simulink model "LIPModel"  (R2016b)
settings: Solver=FixedStepAuto  StartTime=0.0  StopTime=80  FixedStep=0.02  RelTol=1e-3  EnableMultiTasking=on
libraries: powerlib_meascontrol x2
settings Model: Creator=mdai3  LastModifiedBy=WZE7470
settings DataIOCC: ReturnWorkspaceOutputs=on
settings SFSimCC: SimUseLocalCustomCode=on
settings RTWCC: RTWUseLocalCustomCode=on

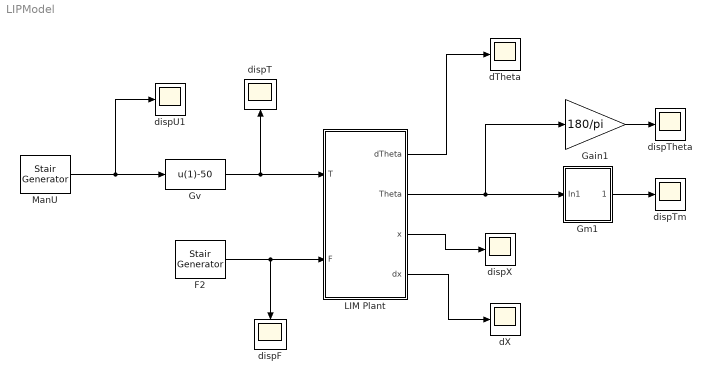
== system LIPModel ==
  F2 : powerlib_meascontrol/Pulse & Signal Generators/Stair Generator  t=[0, 5, 35, 65]  e=[0, 5, -5, 0]  Ts=0
  Gain1 : Gain  Gain=180/pi
  Gm1 : Subsystem  mask(TF with U0, Y0){Num=[1], Den=[0.2 1], U0=-pi/2, Y0=-pi/2}
      mask help: TF with Initial U0, Y0
      mask Display: dpoly(Num,Den,'s');
  Gv : Fcn  Expr=u(1)-50
  LIM Plant : Subsystem  mask(LIP Model){x0=0, Theta0=-pi/2}
      mask prompts: x0 "Initial Position, x0"; Theta0 "Initial Angle"
  ManU : powerlib_meascontrol/Pulse & Signal Generators/Stair Generator  t=[0, 10, 15, 20]  e=[50, 51, 49, 50]  Ts=0
  dTheta : Scope
  dX : Scope
  dispF : Scope
  dispT : Scope
  dispTheta : Scope
  dispTm : Scope
  dispU1 : Scope
  dispX : Scope
  wires:
  ManU/1 -> dispU1/1, Gv/1
  F2/1 -> LIM Plant/2(F), dispF/1
  Gain1/1 -> dispTheta/1
  LIM Plant/2(Theta) -> Gm1/1(In1), Gain1/1
  Gv/1 -> dispT/1, LIM Plant/1(T)
  LIM Plant/1(dTheta) -> dTheta/1
  LIM Plant/3(x) -> dispX/1
  LIM Plant/4(dx) -> dX/1
  Gm1/1(Out1) -> dispTm/1

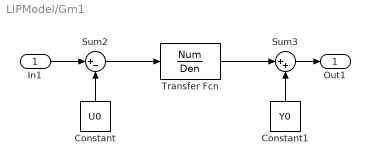
== system LIPModel/Gm1 ==
  In1 : Inport
  Constant : Constant  Value=U0
  Constant1 : Constant  Value=Y0
  Sum2 : Sum  Inputs=|+-  SaturateOnIntegerOverflow=on
  Sum3 : Sum  Inputs=|++  SaturateOnIntegerOverflow=on
  Transfer Fcn : TransferFcn  Numerator=Num  Denominator=Den
  Out1 : Outport
  wires:
  Constant/1 -> Sum2/2
  Constant1/1 -> Sum3/2
  Transfer Fcn/1 -> Sum3/1
  In1/1 -> Sum2/1
  Sum3/1 -> Out1/1
  Sum2/1 -> Transfer Fcn/1

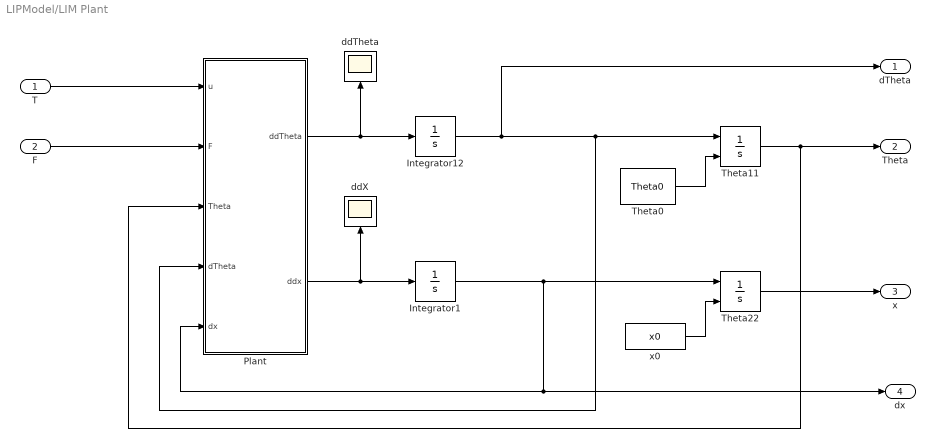
== system LIPModel/LIM Plant ==
  T : Inport
  F : Inport  Port=2
  Integrator1 : Integrator  UpperSaturationLimit=1  LowerSaturationLimit=-1
  Integrator12 : Integrator  UpperSaturationLimit=1  LowerSaturationLimit=-1
  Plant : MATLAB Function  TreatAsAtomicUnit=on
  Theta0 : Constant  Value=Theta0
  Theta11 : Integrator  InitialConditionSource=external  LimitOutput=on  UpperSaturationLimit=pi  LowerSaturationLimit=-pi
  Theta22 : Integrator  InitialConditionSource=external  LimitOutput=on  LowerSaturationLimit=0
  ddTheta : Scope
  ddX : Scope
  x0 : Constant  Value=x0
  dTheta : Outport
  Theta : Outport  Port=2
  x : Outport  Port=3
  dx : Outport  Port=4
  wires:
  F/1 -> Plant/2(F)
  T/1 -> Plant/1(u)
  x0/1 -> Theta22/2
  Theta0/1 -> Theta11/2
  Integrator12/1 -> dTheta/1, Plant/4(dTheta), Theta11/1
  Plant/2(ddx) -> Integrator1/1, ddX/1
  Theta22/1 -> x/1
  Plant/1(ddTheta) -> Integrator12/1, ddTheta/1
  Theta11/1 -> Plant/3(Theta), Theta/1
  Integrator1/1 -> dx/1, Plant/5(dx), Theta22/1

== matlab function LIPModel/LIM Plant/Plant ==
  data: u input; ddTheta output; F input; Theta input; dTheta input; dx input; ddx output
function [ddTheta,ddx] = LIPM(u,F,Theta,dTheta,dx)

%% M*dd + V + G = tau

    %% constant property of model
    m1 = 100; m2 = 1;     
    L = 0.5;    
    g = 9.81;
    
    %% second order state parameter matrix
    % Lagrangian Theta1
    M11 = (m1+m2);
    M12 = -0.5*m2*L*sin(Theta);
    M21 = M12;
    M22 = 1/3*m2*L*L;
        
    M = [M11 M12;
         M21 M22];
    
 %% first order derivative V
    dTheta_sqrt = [dx^2 dTheta^2]';
    matV = zeros(2);
    matV(1,2) = -0.5*m2*L*cos(Theta);
    
    V =  matV * dTheta_sqrt;
    
    %% Gravity term
    G = zeros(2,1);
    G(2) = 1/2*m2*g*L*cos(Theta);
    
    T = [F;u]; 
    fTemp = inv(M)*(T-V-G);
    ddx = fTemp(1)
    ddTheta = fTemp(2);
end
